simulink model "lab_exercice4"  (R2016a)
settings: Solver=FixedStepDiscrete  StartTime=0.0  StopTime=0.1  FixedStep=1/100000  RelTol=1e-3
libraries: dsparch4 x12, dspsigops x3, dspsrcs4 x2
settings Model: Creator=beac2832  LastModifiedBy=beac2832

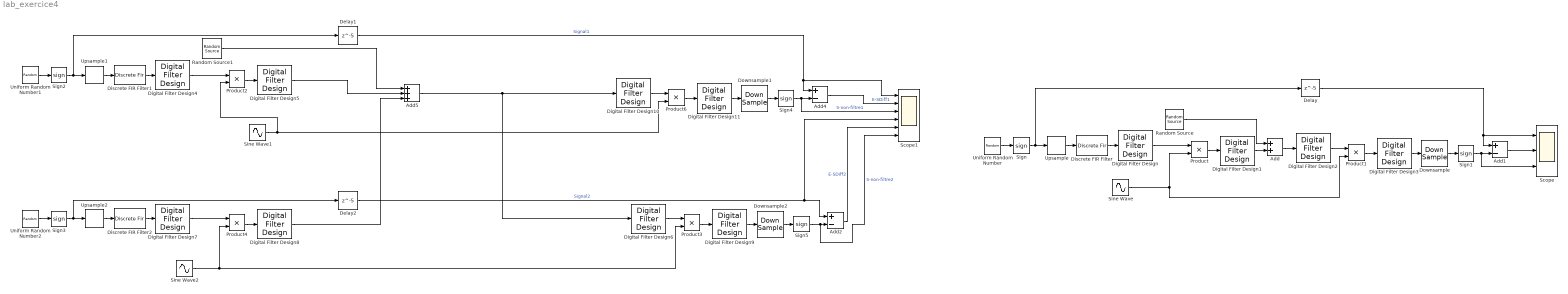
== system lab_exercice4 ==
  Add : Sum
  Add1 : Sum  Inputs=+-
  Add2 : Sum  Inputs=+-
  Add4 : Sum  Inputs=+-
  Add5 : Sum  Inputs=+++
  Delay : Delay  DelayLength=5  InitialCondition=0
  Delay1 : Delay  DelayLength=5  InitialCondition=0
  Delay2 : Delay  DelayLength=5  InitialCondition=0
  Digital Filter Design{,1..11} (12 alike) : dsparch4/Digital Filter Design  mwdsp_browser_bugfix_var=off
  Discrete FIR Filter : DiscreteFir  Coefficients=ones(1,100)
  Discrete FIR Filter1 : DiscreteFir  Coefficients=ones(1,100)
  Discrete FIR Filter2 : DiscreteFir  Coefficients=ones(1,100)
  Downsample : DownSample  N=100  phase=50  RateOptions=Allow multirate processing
  Downsample1 : DownSample  N=100  phase=50  RateOptions=Allow multirate processing
  Downsample2 : DownSample  N=100  phase=50  RateOptions=Allow multirate processing
  Product{,1..4,6} (6 alike) : Product
  Random Source : dspsrcs4/Random Source  SrcType=Gaussian  NormMethod=Ziggurat  CltLength=12  MinVal=0  MaxVal=1  MeanVal=0  VarVal=2  RepMode=Not repeatable  rawSeed=1  IsInherit=on  SampMode=Discrete  SampTime=1  SampFrame=1  DataType=Double  OutComplex=Real  OutputFrames=off
  Random Source1 : dspsrcs4/Random Source  SrcType=Gaussian  NormMethod=Ziggurat  CltLength=12  MinVal=0  MaxVal=1  MeanVal=0  VarVal=2  RepMode=Not repeatable  rawSeed=1  IsInherit=on  SampMode=Discrete  SampTime=1  SampFrame=1  DataType=Double  OutComplex=Real  OutputFrames=off
  Scope : Scope  NumInputPorts=3
  Scope1 : Scope  NumInputPorts=6
  Sign{,1..5} (6 alike) : Signum
  Sine Wave : Sin  Frequency=10000*2*pi  SampleTime=1/100000
  Sine Wave1 : Sin  Frequency=10000*2*pi  Phase=pi/2  SampleTime=1/100000
  Sine Wave2 : Sin  Frequency=10000*2*pi  SampleTime=1/100000
  Uniform Random Number : UniformRandomNumber  SampleTime=1/1000
  Uniform Random Number1 : UniformRandomNumber  SampleTime=1/1000
  Uniform Random Number2 : UniformRandomNumber  SampleTime=1/1000
  Upsample : dspsigops/Upsample  N=100  phase=0  RateOptions=Allow multirate processing  ic=0  mode=Unused parameter value
  Upsample1 : dspsigops/Upsample  N=100  phase=0  RateOptions=Allow multirate processing  ic=0  mode=Unused parameter value
  Upsample2 : dspsigops/Upsample  N=100  phase=0  RateOptions=Allow multirate processing  ic=0  mode=Unused parameter value
  wires:
  Uniform Random Number/1 -> Sign/1
  Sign/1 -> Delay/1, Upsample/1
  Upsample/1 -> Discrete FIR Filter/1
  Discrete FIR Filter/1 -> Digital Filter Design/1
  Digital Filter Design/1 -> Product/1
  Product/1 -> Digital Filter Design1/1
  Digital Filter Design1/1 -> Add/2
  Add/1 -> Digital Filter Design2/1
  Digital Filter Design2/1 -> Product1/1
  Product1/1 -> Digital Filter Design3/1
  Downsample/1 -> Sign1/1
  Digital Filter Design3/1 -> Downsample/1
  Delay/1 -> Scope/1, Add1/1
  Add1/1 -> Scope/2
  Sign1/1 -> Scope/3, Add1/2
  Random Source/1 -> Add/1
  Uniform Random Number1/1 -> Sign2/1
  Sign2/1 -> Delay1/1, Upsample1/1
  Upsample1/1 -> Discrete FIR Filter1/1
  Discrete FIR Filter1/1 -> Digital Filter Design4/1
  Digital Filter Design4/1 -> Product2/1
  Sine Wave/1 -> Product1/2, Product/2
  Product2/1 -> Digital Filter Design5/1
  Uniform Random Number2/1 -> Sign3/1
  Sign3/1 -> Delay2/1, Upsample2/1
  Upsample2/1 -> Discrete FIR Filter2/1
  Discrete FIR Filter2/1 -> Digital Filter Design7/1
  Digital Filter Design7/1 -> Product4/1
  Product4/1 -> Digital Filter Design8/1
  Digital Filter Design10/1 -> Product6/1
  Product6/1 -> Digital Filter Design11/1
  Downsample1/1 -> Sign4/1
  Digital Filter Design11/1 -> Downsample1/1
  Delay1/1 -> Scope1/1, Add4/1  "Signal1"
  Add4/1 -> Scope1/2  "E-SDiff1"
  Sign4/1 -> Scope1/3, Add4/2  "S-non-filtre1"
  Sine Wave1/1 -> Product6/2, Product2/2
  Digital Filter Design8/1 -> Add5/3
  Digital Filter Design5/1 -> Add5/2
  Random Source1/1 -> Add5/1
  Add5/1 -> Digital Filter Design6/1, Digital Filter Design10/1
  Digital Filter Design6/1 -> Product3/1
  Product3/1 -> Digital Filter Design9/1
  Downsample2/1 -> Sign5/1
  Digital Filter Design9/1 -> Downsample2/1
  Delay2/1 -> Scope1/4, Add2/1  "Signal2"
  Sign5/1 -> Scope1/6, Add2/2  "S-non-filtre2"
  Sine Wave2/1 -> Product4/2, Product3/2
  Add2/1 -> Scope1/5  "E-SDiff2"
